simulink model "Ex4_1_P1"  (R2019a)
settings: Solver=VariableStepAuto  StartTime=0.0  StopTime=10.0  RelTol=1e-3
settings Model: Creator=john  LastModifiedBy=john

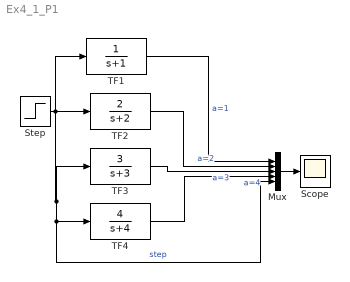
== system Ex4_1_P1 ==
  Mux : Mux  Inputs=5
  Scope : Scope
  Step : Step  SampleTime=0
  TF1 : TransferFcn  Denominator=[1 1]
  TF2 : TransferFcn  Numerator=[2]  Denominator=[1 2]
  TF3 : TransferFcn  Numerator=[3]  Denominator=[1 3]
  TF4 : TransferFcn  Numerator=[4]  Denominator=[1 4]
  wires:
  Step/1 -> Mux/5, TF4/1, TF3/1, TF2/1, TF1/1  "step"
  Mux/1 -> Scope/1
  TF1/1 -> Mux/1  "a=1"
  TF2/1 -> Mux/2  "a=2"
  TF3/1 -> Mux/3  "a=3"
  TF4/1 -> Mux/4  "a=4"
